simulink model "main_v2"  (R2022a)
settings: Solver=VariableStepAuto  StartTime=0.0  StopTime=10.0  RelTol=1e-3
model workspace (MATLAB code in the model file):
  | g = 9.81; % m/s^2
  | L = [240 800 1050 1175 225 200 235 248]/1000; % m
  | 
  | % note from here on L7 does not exist
  | W = [0 0 0 150 200 100 0 50]; % weights
  | I = [0 0 0; 0 0 0; 0 0 0; 2 3 2; 1 18 18; 0.5 2 2; 0 0 0; 1 1 1;]; % Inertia
  | 
  | L5_w = (L(5)*(16/9));
  | 
  | L1 = [300 800]/1000;
  | L2 = [800 300]/1000;
  | L2_w = 480/1000;
  | 
  | arm_width=0.1;
  | 
  | M1 = [150 500];
  | M2 = 750;
  | M3 = [250 50];
  | M4 = 200;
  | M5 = 150;
  | M6 = 100;
  | M7 = 50;
  | 
  | mMIL1 = [0.5 8 8; 10 10 10;];
  | mMIL2 = [50 50 50];
  | mMIL3 = [1 20 20; 0.2 1 1;];
  | mMIL4 = [1 18 18];
  | mMIL5 = [2 3 2];
  | mMIL6 = [0.5 2 2];
  | mMIL7 = [1 1 1];
  | 
  | CB = 300/1000; % m
  | 
  | L0 = 750/1000; %m
  | k = 750*1000; %N/m
  | 
  | P1 = [2000 500 1600];
  | P2 = [2000 -500 1600];
  | P3 = [1600 500 900];
  | P4 = [1600 0 900];
  | P5 = P1;
  | P = [P1; P2; P3; P4; P5;]/1000; % m
  | 
  | Km = [0.5 1.0 1.5]; % Nm/A
  | KmCost = [1 1.25 1.5];
  | J = 0.002; %kgm^2
  | IMax = 16;
  | 
  | KmMax = Km * IMax;
  | 
  | gearboxRatios = [20 50 100 200];
  | gearboxRatioCosts = [1 1.25 1.5 2.5];
undefined symbols (not defined in the file or in its folder): X, Y, Z
libraries: sm_lib x52, fl_lib x8, nesl_utility x7, ee_lib x4, batteryecm_lib x1
(part 2 of 2)

== matlab function main_v2/MATLAB Function ==
  data: x output; t input; y output; z output
function [x,y,z] = fcn(t)
x=2; 
y=0.5; 
z=1.6;
end
